simulink library "GFL_Lib"  (R2019b)
settings: Solver=VariableStepAuto  StartTime=0.0  StopTime=10.0  RelTol=1e-3
undefined symbols (not defined in the file or in its folder): Carm, Diff_CC_ki, Diff_CC_kp, fb, Ib2, Idcb, Ki_i, Ki_Wdiff_pu, Ki_Wtot_pu, Kp_i, Kp_Rvi_pu, Kp_Wdiff_pu, Kp_Wtot_pu, Lb, Lc_eq, Lc_pu, Lf_pu, Sb, Solver_Time_Step, Time_Step, Va0, Vb0, Vb1, Vb2, Vc0, Vdcb, Vm0, Vm0_d, Vm0_q, VSC01_id0, Vvsc0, wb, Zb
libraries: powerlib x90, Control_Lib x57, spsCurrentMeasurementLib x7, simulink x7, spsControlledCurrentSourceLib x6, $bdroot x5, Source_Lib x2, eeGeneralControl x2, powerlib_meascontrol x2, GFo_Lib x1
(part 2 of 5)

== system GFL_Lib/GFL IDEAL VSC ==
  note: do not modify this part if you use the update loaflow script
  note: Common Inputs
  note: Power part
  note: Measurements and normalization
  note: Control part
  dP_set (pu) : Inport
  dQ_set (pu) : Inport  Port=2
  1/Ib2 : Gain  Gain=1/Vb2
  1/Ib3 : Gain  Gain=1/Ib2
  Add : Sum
  Add1 : Sum
  Bridge_Model : Subsystem
  Bus01 : powerlib/Measurements/Three-Phase V-I Measurement  VoltageMeasurement=phase-to-ground  SetLabelV=off  LabelV=Vabc  Vpu=off  VpuLL=off  CurrentMeasurement=yes  SetLabelI=off  LabelI=Iabc  Ipu=off  Pbase=100e6  Vbase=500e3  OutputType=Complex  PhasorSimulation=off  PSBequivalent=0
  Control loops : Subsystem
  DC_Link : Source_Lib/DC_Link  Udc=Udcn  Pb=Pn  H_DC=H_DC
      settings: SourceProductName=VSC4SPS
  Output_Transformer : powerlib/Elements/Three-Phase Transformer (Two Windings)  Winding1Connection=Yg  Winding2Connection=Yg  CoreType=Three single-phase transformers  SetSaturation=off  Hysteresis=off  DataFile='hysteresis'  SetInitialFlux=off  Measurements=None  UNITS=pu  NominalPower=[Sn , fb]  Winding1=[Un1 , Rt_pu/2*(m^2), Lt_pu/2*(m^2)]  Winding2="[Un2*m ,  Rt_pu/2*(m^2), Lt_pu/2*(m^2)]"  Rm=Rm_pu  Lm=Lm_pu  L0=0.5  Saturation=[ 0,0 ; 0.0024,1.2 ; 1.0,1.52 ]  InitialFluxes=[ 0.8 , -0.8 , 0.7 ]  BreakLoop=off  DiscreteSolver=Trapezoidal iterative  DataType=off  TransfoNumber=1
  Pinit : Constant  Value=P0
  Source_For_LF : powerlib/Electrical Sources/Three-Phase Source  Commented=on  InternalConnection=Yg  VoltagePhases=off  Voltage=(690)*0.999921  PhaseAngle=3.7838  Voltage_phases=[25e3 25e3 25e3]/sqrt(3)  PhaseAngles_phases=[0 -120 +120]  Frequency=fb  NonIdealSource=off  SpecifyImpedance=off  Resistance=0  Inductance=0  ShortCircuitLevel=100e6  BaseVoltage=Un  XRratio=7  BusType=PQ  Pref=P0*Sb  Qref=Q0*Sb  Prefabc=[10e3, 10e3, 10e3]  Qrefabc=[0, 0, 0]  Qmin=-inf  Qmax=inf
  Transport Delay1 : TransportDelay  DelayTime=Output_Delay  InitialOutput=[Va0 Vb0 Vc0]
  Vvsc_init : Constant  Value=Q0
  mp3 : Gain  Gain=Vb1
  A : PMIOPort  Side=Right
  B : PMIOPort  Port=2  Side=Right
  C : PMIOPort  Port=3  Side=Right
  + : PMIOPort  Port=4  Side=Left
  - : PMIOPort  Port=5  Side=Left
  m : Outport  VectorParamsAs1DForOutWhenUnconnected=off
  wires:
  Bus01/2 -> [ig_meas]
  Transport Delay1/1 -> Bridge_Model/1(Uref)
  Bus01/1 -> [vg_meas]
  Add/1 -> Control loops/1(P_set)
  Control loops/2(m) -> m/1  "Control"
  mp3/1 -> Transport Delay1/1
  1/Ib3/1 -> Control loops/4(ig_abc_pu)  "ig_pu"
  1/Ib2/1 -> Control loops/3(vg_abc_pu)  "vg_pu"
  [vg_meas] -> 1/Ib2/1
  Control loops/1(vm_abc_ref_pu) -> mp3/1
  Add1/1 -> Control loops/2(Q_set)
  dP_set (pu)/1 -> Add/1
  Pinit/1 -> Add/2
  Vvsc_init/1 -> Add1/2
  dQ_set (pu)/1 -> Add1/1
  [ig_meas] -> 1/Ib3/1
  connections:
  Bridge_Model/LConn2 -- DC_Link/RConn3 -- -/RConn1
  Bridge_Model/LConn1 -- DC_Link/RConn1 -- +/RConn1
  Output_Transformer/RConn3 -- Bus01/LConn3
  Output_Transformer/LConn2 -- Bridge_Model/RConn2
  Output_Transformer/RConn1 -- Bus01/LConn1
  Output_Transformer/RConn2 -- Bus01/LConn2
  Output_Transformer/LConn1 -- Bridge_Model/RConn1
  Output_Transformer/LConn3 -- Bridge_Model/RConn3
  Bus01/RConn1 -- Source_For_LF/RConn1 -- A/RConn1
  Bus01/RConn3 -- Source_For_LF/RConn3 -- C/RConn1
  Bus01/RConn2 -- Source_For_LF/RConn2 -- B/RConn1

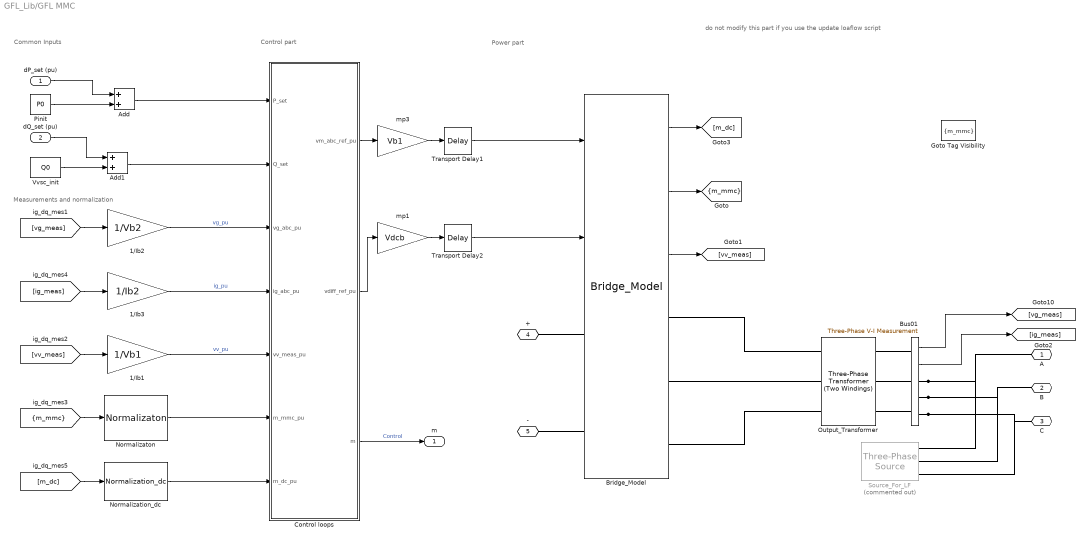
== system GFL_Lib/GFL MMC ==
  note: Common Inputs
  note: Control part
  note: Power part
  note: do not modify this part if you use the update loaflow script
  note: Measurements and normalization
  dP_set (pu) : Inport
  dQ_set (pu) : Inport  Port=2
  1/Ib1 : Gain  Gain=1/Vb1
  1/Ib2 : Gain  Gain=1/Vb2
  1/Ib3 : Gain  Gain=1/Ib2
  Add : Sum
  Add1 : Sum
  Bridge_Model : $bdroot/GFM_VC MMC/Bridge_Model  SystemSampleTime=-1  Latency=0  AutoFrameSizeCalculation=off
  Bus01 : powerlib/Measurements/Three-Phase V-I Measurement  VoltageMeasurement=phase-to-ground  SetLabelV=off  LabelV=Vabc  Vpu=off  VpuLL=off  CurrentMeasurement=yes  SetLabelI=off  LabelI=Iabc  Ipu=off  Pbase=100e6  Vbase=500e3  OutputType=Complex  PhasorSimulation=off  PSBequivalent=0
  Control loops : Subsystem
  Goto Tag Visibility : GotoTagVisibility  GotoTag=m_mmc
  Normalization_dc : $bdroot/GFM_VC MMC/Normalization_dc  SystemSampleTime=-1  Latency=0  AutoFrameSizeCalculation=off
  Normalizaton : $bdroot/GFM_VC MMC/Normalizaton  SystemSampleTime=-1  Latency=0  AutoFrameSizeCalculation=off
  Output_Transformer : powerlib/Elements/Three-Phase Transformer (Two Windings)  Winding1Connection=Yg  Winding2Connection=Yg  CoreType=Three single-phase transformers  SetSaturation=off  Hysteresis=off  DataFile='hysteresis'  SetInitialFlux=off  Measurements=None  UNITS=pu  NominalPower=[Sn , fb]  Winding1=[Un1 , Rt_pu/2 , Lt_pu/2]  Winding2=[Un2 , Rt_pu/2 , Lt_pu/2]  Rm=Rm_pu  Lm=Lm_pu  L0=0.5  Saturation=[ 0,0 ; 0.0024,1.2 ; 1.0,1.52 ]  InitialFluxes=[ 0.8 , -0.8 , 0.7 ]  BreakLoop=off  DiscreteSolver=Trapezoidal iterative  DataType=off  TransfoNumber=1
  Pinit : Constant  Value=P0
  Source_For_LF : powerlib/Electrical Sources/Three-Phase Source  Commented=on  InternalConnection=Yg  VoltagePhases=off  Voltage=(400000)*1  PhaseAngle=9.4519e-16  Voltage_phases=[25e3 25e3 25e3]/sqrt(3)  PhaseAngles_phases=[0 -120 +120]  Frequency=fb  NonIdealSource=off  SpecifyImpedance=off  Resistance=0  Inductance=0  ShortCircuitLevel=100e6  BaseVoltage=Un  XRratio=7  BusType=PQ  Pref=P0*Sb  Qref=Q0*Sb  Prefabc=[10e3, 10e3, 10e3]  Qrefabc=[0, 0, 0]  Qmin=-inf  Qmax=inf
  Transport Delay1 : TransportDelay  DelayTime=Output_Delay  InitialOutput=[Va0 Vb0 Vc0]
  Transport Delay2 : TransportDelay  DelayTime=Output_Delay  InitialOutput=[Udcn/2 Udcn/2 Udcn/2]
  Vvsc_init : Constant  Value=Q0
  mp1 : Gain  Gain=Vdcb
  mp3 : Gain  Gain=Vb1
  A : PMIOPort  Side=Right
  B : PMIOPort  Port=2  Side=Right
  C : PMIOPort  Port=3  Side=Right
  + : PMIOPort  Port=4  Side=Left
  - : PMIOPort  Port=5  Side=Left
  m : Outport  VectorParamsAs1DForOutWhenUnconnected=off
  tag scope: m_mmc=scoped
  wires:
  Add/1 -> Control loops/1(P_set)
  Control loops/3(m) -> m/1  "Control"
  mp3/1 -> Transport Delay1/1
  Control loops/1(vm_abc_ref_pu) -> mp3/1
  Add1/1 -> Control loops/2(Q_set)
  dP_set (pu)/1 -> Add/1
  Pinit/1 -> Add/2
  Vvsc_init/1 -> Add1/2
  dQ_set (pu)/1 -> Add1/1
  Bridge_Model/2 -> [m_mmc]
  Transport Delay2/1 -> Bridge_Model/2
  Bridge_Model/3 -> [vv_meas]
  Bus01/2 -> [ig_meas]
  Bridge_Model/1 -> [m_dc]
  Bus01/1 -> [vg_meas]
  Transport Delay1/1 -> Bridge_Model/1
  1/Ib1/1 -> Control loops/5(vv_meas_pu)  "vv_pu"
  Normalization_dc/1 -> Control loops/7(m_dc_pu)
  [vg_meas] -> 1/Ib2/1
  Normalizaton/1 -> Control loops/6(m_mmc_pu)
  [m_mmc] -> Normalizaton/1
  [vv_meas] -> 1/Ib1/1
  [ig_meas] -> 1/Ib3/1
  [m_dc] -> Normalization_dc/1
  1/Ib3/1 -> Control loops/4(ig_abc_pu)  "ig_pu"
  1/Ib2/1 -> Control loops/3(vg_abc_pu)  "vg_pu"
  mp1/1 -> Transport Delay2/1
  Control loops/2(vdiff_ref_pu) -> mp1/1
  connections:
  Bus01/RConn3 -- Source_For_LF/RConn3 -- C/RConn1
  Bus01/RConn1 -- Source_For_LF/RConn1 -- A/RConn1
  Bus01/RConn2 -- Source_For_LF/RConn2 -- B/RConn1
  Bridge_Model/RConn2 -- Output_Transformer/LConn2
  Output_Transformer/RConn1 -- Bus01/LConn1
  +/RConn1 -- Bridge_Model/LConn1
  -/RConn1 -- Bridge_Model/LConn2
  Output_Transformer/RConn2 -- Bus01/LConn2
  Bridge_Model/RConn1 -- Output_Transformer/LConn1
  Output_Transformer/RConn3 -- Bus01/LConn3
  Bridge_Model/RConn3 -- Output_Transformer/LConn3

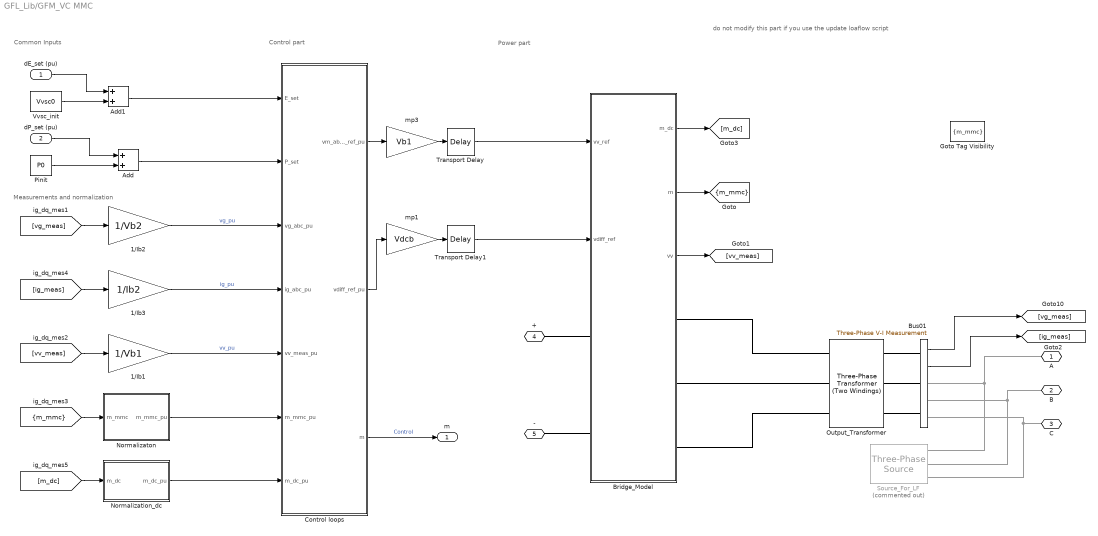
== system GFL_Lib/GFM_VC MMC ==
  note: do not modify this part if you use the update loaflow script
  note: Common Inputs
  note: Power part
  note: Measurements and normalization
  note: Control part
  dE_set (pu) : Inport
  dP_set (pu) : Inport  Port=2
  1/Ib1 : Gain  Gain=1/Vb1
  1/Ib2 : Gain  Gain=1/Vb2
  1/Ib3 : Gain  Gain=1/Ib2
  Add : Sum
  Add1 : Sum
  Bridge_Model : Subsystem
  Bus01 : powerlib/Measurements/Three-Phase V-I Measurement  VoltageMeasurement=phase-to-ground  SetLabelV=off  LabelV=Vabc  Vpu=off  VpuLL=off  CurrentMeasurement=yes  SetLabelI=off  LabelI=Iabc  Ipu=off  Pbase=100e6  Vbase=500e3  OutputType=Complex  PhasorSimulation=off  PSBequivalent=0
  Control loops : Subsystem
  Goto Tag Visibility : GotoTagVisibility  GotoTag=m_mmc
  Normalization_dc : Subsystem
  Normalizaton : Subsystem
  Output_Transformer : powerlib/Elements/Three-Phase Transformer (Two Windings)  Winding1Connection=Yg  Winding2Connection=Yg  CoreType=Three single-phase transformers  SetSaturation=off  Hysteresis=off  DataFile='hysteresis'  SetInitialFlux=off  Measurements=None  UNITS=pu  NominalPower=[Sn , fb]  Winding1=[Un1 , Rt_pu/2 , Lt_pu/2]  Winding2=[Un2 , Rt_pu/2 , Lt_pu/2]  Rm=Rm_pu  Lm=Lm_pu  L0=0.5  Saturation=[ 0,0 ; 0.0024,1.2 ; 1.0,1.52 ]  InitialFluxes=[ 0.8 , -0.8 , 0.7 ]  BreakLoop=off  DiscreteSolver=Trapezoidal iterative  DataType=off  TransfoNumber=1
  Pinit : Constant  Value=P0
  Source_For_LF : powerlib/Electrical Sources/Three-Phase Source  Commented=on  InternalConnection=Yg  VoltagePhases=off  Voltage=(400000)*1  PhaseAngle=9.4519e-16  Voltage_phases=[25e3 25e3 25e3]/sqrt(3)  PhaseAngles_phases=[0 -120 +120]  Frequency=fb  NonIdealSource=off  SpecifyImpedance=off  Resistance=0  Inductance=0  ShortCircuitLevel=100e6  BaseVoltage=Un  XRratio=7  BusType=PQ  Pref=P0*Sb  Qref=Q0*Sb  Prefabc=[10e3, 10e3, 10e3]  Qrefabc=[0, 0, 0]  Qmin=-inf  Qmax=inf
  Transport Delay : TransportDelay  DelayTime=Output_Delay  InitialOutput=[Va0 Vb0 Vc0]
  Transport Delay1 : TransportDelay  DelayTime=Output_Delay  InitialOutput=[Udcn/2 Udcn/2 Udcn/2]
  Vvsc_init : Constant  Value=Vvsc0
  mp1 : Gain  Gain=Vdcb
  mp3 : Gain  Gain=Vb1
  A : PMIOPort  Side=Right
  B : PMIOPort  Port=2  Side=Right
  C : PMIOPort  Port=3  Side=Right
  + : PMIOPort  Port=4  Side=Left
  - : PMIOPort  Port=5  Side=Left
  m : Outport  VectorParamsAs1DForOutWhenUnconnected=off
  tag scope: m_mmc=scoped
  wires:
  Add/1 -> Control loops/2(P_set)
  Control loops/3(m) -> m/1  "Control"
  mp3/1 -> Transport Delay/1
  1/Ib3/1 -> Control loops/4(ig_abc_pu)  "ig_pu"
  1/Ib2/1 -> Control loops/3(vg_abc_pu)  "vg_pu"
  [vg_meas] -> 1/Ib2/1
  Control loops/1(vm_abc_ref_pu) -> mp3/1
  Add1/1 -> Control loops/1(E_set)
  Transport Delay/1 -> Bridge_Model/1(vv_ref)
  dP_set (pu)/1 -> Add/1
  Pinit/1 -> Add/2
  Vvsc_init/1 -> Add1/2
  Bus01/1 -> [vg_meas]
  dE_set (pu)/1 -> Add1/1
  Bus01/2 -> [ig_meas]
  [ig_meas] -> 1/Ib3/1
  Control loops/2(vdiff_ref_pu) -> mp1/1
  mp1/1 -> Transport Delay1/1
  Transport Delay1/1 -> Bridge_Model/2(vdiff_ref)
  Bridge_Model/3(vv) -> [vv_meas]
  [vv_meas] -> 1/Ib1/1
  1/Ib1/1 -> Control loops/5(vv_meas_pu)  "vv_pu"
  [m_mmc] -> Normalizaton/1(m_mmc)
  Normalizaton/1(m_mmc_pu) -> Control loops/6(m_mmc_pu)
  Bridge_Model/1(m_dc) -> [m_dc]
  Normalization_dc/1(m_dc_pu) -> Control loops/7(m_dc_pu)
  [m_dc] -> Normalization_dc/1(m_dc)
  Bridge_Model/2(m) -> [m_mmc]
  connections:
  Output_Transformer/RConn1 -- Bus01/LConn1
  Output_Transformer/RConn2 -- Bus01/LConn2
  Output_Transformer/RConn3 -- Bus01/LConn3
  Source_For_LF/RConn2 -- B/RConn1 -- Bus01/RConn2
  Source_For_LF/RConn1 -- A/RConn1 -- Bus01/RConn1
  Source_For_LF/RConn3 -- C/RConn1 -- Bus01/RConn3
  Bridge_Model/RConn1 -- Output_Transformer/LConn1
  Bridge_Model/RConn2 -- Output_Transformer/LConn2
  Bridge_Model/RConn3 -- Output_Transformer/LConn3
  +/RConn1 -- Bridge_Model/LConn1
  -/RConn1 -- Bridge_Model/LConn2

== system GFL_Lib/Mean Model 2-Level L-filter with DC Link ==
  note: Control part
  note: Measurements and normalization
  note: Power part
  note: Common Inputs
  note: do not modify this part if you use the update loaflow script
  dP_set (pu) : Inport
  dQ_set (pu) : Inport  Port=2
  1/Ib2 : Gain  Gain=1/Vb2
  1/Ib3 : Gain  Gain=1/Ib2
  Add : Sum
  Add1 : Sum
  Bridge_Model : Subsystem
  Bus01 : powerlib/Measurements/Three-Phase V-I Measurement  VoltageMeasurement=phase-to-ground  SetLabelV=off  LabelV=Vabc  Vpu=off  VpuLL=off  CurrentMeasurement=yes  SetLabelI=off  LabelI=Iabc  Ipu=off  Pbase=100e6  Vbase=500e3  OutputType=Complex  PhasorSimulation=off  PSBequivalent=0
  Control loops : Subsystem
  DC_Link_1 : powerlib/Elements/Series RLC Branch  LConnTagsString=__new0  RConnTagsString=__new0  BranchType=C  Resistance=1  Inductance=1e-3  SetiL0=off  InitialCurrent=0  Capacitance=0.00039063  Setx0=on  InitialVoltage=Udcn/2  Measurements=None
  DC_Link_2 : powerlib/Elements/Series RLC Branch  LConnTagsString=__new0  RConnTagsString=__new0  BranchType=C  Resistance=1  Inductance=1e-3  SetiL0=off  InitialCurrent=0  Capacitance=0.00039063  Setx0=on  InitialVoltage=Udcn/2  Measurements=None
  Delay : Delay  DelayLength=1  InitialCondition=[Va0 Vb0 Vc0]  SampleTime=Solver_Time_Step
  Ground : powerlib/Elements/Ground  LConnTagsString=a
  Output_Transformer : powerlib/Elements/Three-Phase Transformer (Two Windings)  Winding1Connection=Yg  Winding2Connection=Yg  CoreType=Three single-phase transformers  SetSaturation=off  Hysteresis=off  DataFile='hysteresis'  SetInitialFlux=off  Measurements=None  UNITS=pu  NominalPower=[Sn , fb]  Winding1=[Un1 , Rt_pu/2*(m^2), Lt_pu/2*(m^2)]  Winding2="[Un2*m ,  Rt_pu/2*(m^2), Lt_pu/2*(m^2)]"  Rm=Rm_pu  Lm=Lm_pu  L0=0.5  Saturation=[ 0,0 ; 0.0024,1.2 ; 1.0,1.52 ]  InitialFluxes=[ 0.8 , -0.8 , 0.7 ]  BreakLoop=off  DiscreteSolver=Trapezoidal iterative  DataType=off  TransfoNumber=1
  Pinit : Constant  Value=P0
  Source_For_LF : powerlib/Electrical Sources/Three-Phase Source  Commented=on  InternalConnection=Yg  VoltagePhases=off  Voltage=(400000)*1.01081  PhaseAngle=0.4912  Voltage_phases=[25e3 25e3 25e3]/sqrt(3)  PhaseAngles_phases=[0 -120 +120]  Frequency=fb  NonIdealSource=off  SpecifyImpedance=off  Resistance=0  Inductance=0  ShortCircuitLevel=100e6  BaseVoltage=Un  XRratio=7  BusType=PQ  Pref=P0*Sb  Qref=Q0*Sb  Prefabc=[10e3, 10e3, 10e3]  Qrefabc=[0, 0, 0]  Qmin=-inf  Qmax=inf
  Vvsc_init : Constant  Value=Q0
  mp3 : Gain  Gain=Vb1
  A : PMIOPort  Side=Right
  B : PMIOPort  Port=2  Side=Right
  C : PMIOPort  Port=3  Side=Right
  A1 : PMIOPort  Port=4  Side=Left
  A2 : PMIOPort  Port=5  Side=Left
  m : Outport  VectorParamsAs1DForOutWhenUnconnected=off
  wires:
  [ig_meas] -> 1/Ib3/1
  dQ_set (pu)/1 -> Add1/1
  Vvsc_init/1 -> Add1/2
  Pinit/1 -> Add/2
  dP_set (pu)/1 -> Add/1
  Add1/1 -> Control loops/2(Q_set)
  Control loops/1(vm_abc_ref_pu) -> mp3/1
  [vg_meas] -> 1/Ib2/1
  1/Ib2/1 -> Control loops/3(vg_abc_pu)  "vg_pu"
  1/Ib3/1 -> Control loops/4(ig_abc_pu)  "ig_pu"
  mp3/1 -> Delay/1
  Control loops/2(m) -> m/1  "Control"
  Add/1 -> Control loops/1(P_set)
  Bus01/1 -> [vg_meas]
  Delay/1 -> Bridge_Model/1(Uref)
  Bus01/2 -> [ig_meas]
  connections:
  B/RConn1 -- Source_For_LF/RConn2 -- Bus01/RConn2
  C/RConn1 -- Source_For_LF/RConn3 -- Bus01/RConn3
  A/RConn1 -- Source_For_LF/RConn1 -- Bus01/RConn1
  Output_Transformer/LConn3 -- Bridge_Model/RConn3
  Output_Transformer/LConn1 -- Bridge_Model/RConn1
  Output_Transformer/RConn2 -- Bus01/LConn2
  Output_Transformer/RConn1 -- Bus01/LConn1
  Output_Transformer/LConn2 -- Bridge_Model/RConn2
  Output_Transformer/RConn3 -- Bus01/LConn3
  DC_Link_1/LConn1 -- A1/RConn1 -- Bridge_Model/LConn1
  DC_Link_2/RConn1 -- Bridge_Model/LConn2 -- A2/RConn1
  DC_Link_1/RConn1 -- DC_Link_2/LConn1 -- Ground/LConn1

== system GFL_Lib/Mean Model 2-Level L-filter_old ==
  note: Control part
  note: Measurements and normalization
  note: Power part
  note: Common Inputs
  note: do not modify this part if you use the update loaflow script
  dP_set (pu) : Inport
  dQ_set (pu) : Inport  Port=2
  1/Ib2 : Gain  Gain=1/Vb2
  1/Ib3 : Gain  Gain=1/Ib2
  Add : Sum
  Add1 : Sum
  Bridge_Model : Subsystem
  Bus01 : powerlib/Measurements/Three-Phase V-I Measurement  VoltageMeasurement=phase-to-ground  SetLabelV=off  LabelV=Vabc  Vpu=off  VpuLL=off  CurrentMeasurement=yes  SetLabelI=off  LabelI=Iabc  Ipu=off  Pbase=100e6  Vbase=500e3  OutputType=Complex  PhasorSimulation=off  PSBequivalent=0
  Control loops : Subsystem
  DC_Link : Source_Lib/DC_Link  Udc=Udcn  Pb=Pn  H_DC=H_DC
      settings: SourceProductName=VSC4SPS
  Delay : Delay  DelayLength=1  InitialCondition=[Va0 Vb0 Vc0]  SampleTime=Output_Delay/1.5
  Output_Transformer : powerlib/Elements/Three-Phase Transformer (Two Windings)  Winding1Connection=Yg  Winding2Connection=Yg  CoreType=Three single-phase transformers  SetSaturation=off  Hysteresis=off  DataFile='hysteresis'  SetInitialFlux=off  Measurements=None  UNITS=pu  NominalPower=[Sn , fb]  Winding1=[Un1 , Rt_pu/2*(m^2), Lt_pu/2*(m^2)]  Winding2="[Un2*m ,  Rt_pu/2*(m^2), Lt_pu/2*(m^2)]"  Rm=Rm_pu  Lm=Lm_pu  L0=0.5  Saturation=[ 0,0 ; 0.0024,1.2 ; 1.0,1.52 ]  InitialFluxes=[ 0.8 , -0.8 , 0.7 ]  BreakLoop=off  DiscreteSolver=Trapezoidal iterative  DataType=off  TransfoNumber=1
  Pinit : Constant  Value=P0
  Source_For_LF : powerlib/Electrical Sources/Three-Phase Source  Commented=on  InternalConnection=Yg  VoltagePhases=off  Voltage=(400000)*1.01081  PhaseAngle=0.4912  Voltage_phases=[25e3 25e3 25e3]/sqrt(3)  PhaseAngles_phases=[0 -120 +120]  Frequency=fb  NonIdealSource=off  SpecifyImpedance=off  Resistance=0  Inductance=0  ShortCircuitLevel=100e6  BaseVoltage=Un  XRratio=7  BusType=PQ  Pref=P0*Sb  Qref=Q0*Sb  Prefabc=[10e3, 10e3, 10e3]  Qrefabc=[0, 0, 0]  Qmin=-inf  Qmax=inf
  Vvsc_init : Constant  Value=Q0
  mp3 : Gain  Gain=Vb1
  A : PMIOPort  Side=Right
  B : PMIOPort  Port=2  Side=Right
  C : PMIOPort  Port=3  Side=Right
  + : PMIOPort  Port=4  Side=Left
  0 : PMIOPort  Port=5  Side=Left
  - : PMIOPort  Port=6  Side=Left
  m : Outport  VectorParamsAs1DForOutWhenUnconnected=off
  wires:
  [ig_meas] -> 1/Ib3/1
  dQ_set (pu)/1 -> Add1/1
  Vvsc_init/1 -> Add1/2
  Pinit/1 -> Add/2
  dP_set (pu)/1 -> Add/1
  Add1/1 -> Control loops/2(Q_set)
  Control loops/1(vm_abc_ref_pu) -> mp3/1
  [vg_meas] -> 1/Ib2/1
  1/Ib2/1 -> Control loops/3(vg_abc_pu)  "vg_pu"
  1/Ib3/1 -> Control loops/4(ig_abc_pu)  "ig_pu"
  mp3/1 -> Delay/1
  Control loops/2(m) -> m/1  "Control"
  Add/1 -> Control loops/1(P_set)
  Bus01/1 -> [vg_meas]
  Delay/1 -> Bridge_Model/1(Uref)
  Bus01/2 -> [ig_meas]
  connections:
  B/RConn1 -- Source_For_LF/RConn2 -- Bus01/RConn2
  C/RConn1 -- Source_For_LF/RConn3 -- Bus01/RConn3
  A/RConn1 -- Source_For_LF/RConn1 -- Bus01/RConn1
  Output_Transformer/LConn3 -- Bridge_Model/RConn3
  Output_Transformer/LConn1 -- Bridge_Model/RConn1
  Output_Transformer/RConn2 -- Bus01/LConn2
  Output_Transformer/RConn1 -- Bus01/LConn1
  Output_Transformer/LConn2 -- Bridge_Model/RConn2
  Output_Transformer/RConn3 -- Bus01/LConn3
  DC_Link/RConn1 -- +/RConn1 -- Bridge_Model/LConn1
  DC_Link/RConn3 -- Bridge_Model/LConn2 -- -/RConn1
  0/RConn1 -- DC_Link/RConn2

== system GFL_Lib/Mean Model 2-Level L-filter_sav ==
  note: do not modify this part if you use the update loaflow script
  note: Transformer
  note: Common Inputs
  note: Power part
  note: Measurements and normalization
  note: Control part
  dQ_set (pu) : Inport
  dP_set (pu) : Inport  Port=2
  1/Ib2 : Gain  Gain=1/Vb2
  1/Ib3 : Gain  Gain=1/Ib2
  Add : Sum
  Add1 : Sum
  Bus Creator : BusCreator  Inputs=3
  Bus01 : powerlib/Measurements/Three-Phase V-I Measurement  VoltageMeasurement=phase-to-ground  SetLabelV=off  LabelV=Vabc  Vpu=off  VpuLL=off  CurrentMeasurement=yes  SetLabelI=off  LabelI=Iabc  Ipu=off  Pbase=100e6  Vbase=500e3  OutputType=Complex  PhasorSimulation=off  PSBequivalent=0
  Control loops : Subsystem
  DC Voltage Source : powerlib/Electrical Sources/DC Voltage Source  Amplitude=Udcn  Measurements=Voltage
  Load Flow Bus : powerlib/Measurements/Load Flow Bus  LConnTagsString=a  Phases=single  Connectors=on one side  ID=Mean Model 2-Level L-filter_sav  Vbase=Un2  Vref=1.0015  Vangle=0.56166  VLF=1.002  VLFb=1  VLFc=1  angleLF=0.5617  angleLFb=0  angleLFc=0
  Mean_Model : Subsystem
  Memory1 : Memory  InitialCondition=[Va0 Vb0 Vc0]
  Output_Transformer : powerlib/Elements/Three-Phase Transformer (Two Windings)  Winding1Connection=Yg  Winding2Connection=Yg  CoreType=Three single-phase transformers  SetSaturation=off  Hysteresis=off  DataFile='hysteresis'  SetInitialFlux=off  Measurements=None  UNITS=pu  NominalPower=[Sn , fb]  Winding1=[Un1 , Rt_pu/2 , Lt_pu/2]  Winding2=[Un2 , Rt_pu/2 , Lt_pu/2]  Rm=Rm_pu  Lm=Lm_pu  L0=0.5  Saturation=[ 0,0 ; 0.0024,1.2 ; 1.0,1.52 ]  InitialFluxes=[ 0.8 , -0.8 , 0.7 ]  BreakLoop=off  DiscreteSolver=Trapezoidal iterative  DataType=off  TransfoNumber=1
  Pinit : Constant  Value=P0
  Source_For_LF : powerlib/Electrical Sources/Three-Phase Source  Commented=on  InternalConnection=Yg  VoltagePhases=off  Voltage=(400)*1.00151  PhaseAngle=0.56166  Voltage_phases=[25e3 25e3 25e3]/sqrt(3)  PhaseAngles_phases=[0 -120 +120]  Frequency=fb  NonIdealSource=off  SpecifyImpedance=off  Resistance=0  Inductance=0  ShortCircuitLevel=100e6  BaseVoltage=Un  XRratio=7  BusType=PQ  Pref=P0*Sb  Qref=Q0*Sb  Prefabc=[10e3, 10e3, 10e3]  Qrefabc=[0, 0, 0]  Qmin=-inf  Qmax=inf
  Vvsc_init : Constant  Value=Q0
  mp3 : Gain  Gain=Vb1
  A : PMIOPort  Side=Right
  B : PMIOPort  Port=2  Side=Right
  C : PMIOPort  Port=3  Side=Right
  m : Outport  VectorParamsAs1DForOutWhenUnconnected=off
  wires:
  Add/1 -> Control loops/1(P_set)
  Control loops/2(m) -> Bus Creator/1  "Control"
  mp3/1 -> Memory1/1
  1/Ib3/1 -> Bus Creator/3, Control loops/4(ig_abc_pu)  "ig_pu"
  1/Ib2/1 -> Bus Creator/2, Control loops/3(vg_abc_pu)  "vg_pu"
  Bus Creator/1 -> m/1
  [vg_meas] -> 1/Ib2/1
  Control loops/1(vm_abc_ref_pu) -> mp3/1
  Add1/1 -> Control loops/2(Q_set)
  Memory1/1 -> Mean_Model/1(Uref)
  dP_set (pu)/1 -> Add/1
  Pinit/1 -> Add/2
  Vvsc_init/1 -> Add1/2
  Bus01/1 -> [vg_meas]
  dQ_set (pu)/1 -> Add1/1
  Bus01/2 -> [ig_meas]
  [ig_meas] -> 1/Ib3/1
  connections:
  DC Voltage Source/LConn1 -- Mean_Model/LConn2
  Output_Transformer/RConn1 -- Bus01/LConn1
  Output_Transformer/RConn2 -- Bus01/LConn2
  DC Voltage Source/RConn1 -- Mean_Model/LConn1
  Output_Transformer/RConn3 -- Bus01/LConn3
  Source_For_LF/RConn2 -- B/RConn1 -- Bus01/RConn2
  Mean_Model/RConn1 -- Output_Transformer/LConn1
  Mean_Model/RConn2 -- Output_Transformer/LConn2
  Mean_Model/RConn3 -- Output_Transformer/LConn3
  Source_For_LF/RConn1 -- Load Flow Bus/LConn1 -- A/RConn1 -- Bus01/RConn1
  Source_For_LF/RConn3 -- C/RConn1 -- Bus01/RConn3

== system GFL_Lib/Mean Model 2-Level LCL-filter [under construction] ==
  note: Common Inputs
  note: Power part
  note: Measurements and normalization
  note: Control part
  dQ_set (pu) : Inport
  dP_set (pu) : Inport  Port=2
  1/Ib2 : Gain  Gain=1/Vb2
  1/Ib3 : Gain  Gain=1/Ib2
  Add : Sum
  Add1 : Sum
  Bus Creator : BusCreator  Inputs=3
  Bus01 : powerlib/Measurements/Three-Phase V-I Measurement  VoltageMeasurement=phase-to-ground  SetLabelV=off  LabelV=Vabc  Vpu=off  VpuLL=off  CurrentMeasurement=yes  SetLabelI=off  LabelI=Iabc  Ipu=off  Pbase=100e6  Vbase=500e3  OutputType=Complex  PhasorSimulation=off  PSBequivalent=0
  Bus1 : powerlib/Measurements/Three-Phase V-I Measurement  VoltageMeasurement=phase-to-ground  SetLabelV=off  LabelV=Vabc  Vpu=off  VpuLL=off  CurrentMeasurement=no  SetLabelI=off  LabelI=Iabc  Ipu=off  Pbase=100e6  Vbase=500e3  OutputType=Complex  PhasorSimulation=off  PSBequivalent=0
  Bus2 : powerlib/Measurements/Three-Phase V-I Measurement  VoltageMeasurement=no  SetLabelV=off  LabelV=Vabc  Vpu=off  VpuLL=off  CurrentMeasurement=yes  SetLabelI=off  LabelI=Iabc  Ipu=off  Pbase=100e6  Vbase=500e3  OutputType=Complex  PhasorSimulation=off  PSBequivalent=0
  Control loops : Subsystem
  DC Voltage Source : powerlib/Electrical Sources/DC Voltage Source  Amplitude=Udcn  Measurements=Voltage
  Load Flow Bus : powerlib/Measurements/Load Flow Bus  LConnTagsString=a  Phases=single  Connectors=on one side  ID=|  Vbase=Un2  Vref=1.0015  Vangle=0.56166  VLF=1.002  VLFb=1  VLFc=1  angleLF=0.5617  angleLFb=0  angleLFc=0
      | Mean Model
      | 2-Level LCL-filter [under construction]
  Mean_model : Subsystem
  Memory1 : Memory  InitialCondition=[Va0 Vb0 Vc0]
  Output_Filter : GFo_Lib/Mean Model 2-Level LCL-filter/Output_Filter
      settings: SourceProductName=VSC4SPS
  Output_Transformer : powerlib/Elements/Three-Phase Transformer (Two Windings)  Winding1Connection=Yg  Winding2Connection=Yg  CoreType=Three single-phase transformers  SetSaturation=off  Hysteresis=off  DataFile='hysteresis'  SetInitialFlux=off  Measurements=None  UNITS=pu  NominalPower=[Sn , fb]  Winding1=[Un1 , Rt_pu/2 , Lt_pu/2]  Winding2=[Un2 , Rt_pu/2 , Lt_pu/2]  Rm=Rm_pu  Lm=Lm_pu  L0=0.5  Saturation=[ 0,0 ; 0.0024,1.2 ; 1.0,1.52 ]  InitialFluxes=[-1.0109960716468 0.506091473811006 0.504904597835851]  BreakLoop=off  DiscreteSolver=Trapezoidal iterative  DataType=off  TransfoNumber=1
  Pinit : Constant  Value=P0
  Source_For_LF : powerlib/Electrical Sources/Three-Phase Source  Commented=on  InternalConnection=Yg  VoltagePhases=off  Voltage=(400)*1.00151  PhaseAngle=0.56166  Voltage_phases=[25e3 25e3 25e3]/sqrt(3)  PhaseAngles_phases=[0 -120 +120]  Frequency=fb  NonIdealSource=off  SpecifyImpedance=off  Resistance=0  Inductance=0  ShortCircuitLevel=100e6  BaseVoltage=Un  XRratio=7  BusType=PQ  Pref=P0*Sb  Qref=Q0*Sb  Prefabc=[10e3, 10e3, 10e3]  Qrefabc=[0, 0, 0]  Qmin=-inf  Qmax=inf
  Vvsc_init : Constant  Value=Q0
  mp3 : Gain  Gain=Vb1
  A : PMIOPort  Side=Right
  B : PMIOPort  Port=2  Side=Right
  C : PMIOPort  Port=3  Side=Right
  m : Outport  VectorParamsAs1DForOutWhenUnconnected=off
  wires:
  Add/1 -> Control loops/1(P_set)
  Control loops/2(m) -> Bus Creator/1  "Control"
  mp3/1 -> Memory1/1
  1/Ib3/1 -> Bus Creator/3, Control loops/4(ig_abc_pu)  "ig_pu"
  1/Ib2/1 -> Bus Creator/2, Control loops/3(vg_abc_pu)  "vg_pu"
  Bus Creator/1 -> m/1
  [vg_meas] -> 1/Ib2/1
  Control loops/1(vm_abc_ref_pu) -> mp3/1
  Add1/1 -> Control loops/2(Q_set)
  Memory1/1 -> Mean_model/1(Uref)
  dP_set (pu)/1 -> Add/1
  Pinit/1 -> Add/2
  Vvsc_init/1 -> Add1/2
  Bus01/1 -> [vg_meas]
  dQ_set (pu)/1 -> Add1/1
  Bus01/2 -> [ig_meas]
  [ig_meas] -> 1/Ib3/1
  Bus1/1 -> [eg_meas]
  Bus2/1 -> [is_meas]
  connections:
  DC Voltage Source/LConn1 -- Mean_model/LConn2
  Bus01/LConn1 -- Output_Transformer/RConn1
  Bus01/LConn2 -- Output_Transformer/RConn2
  DC Voltage Source/RConn1 -- Mean_model/LConn1
  Bus01/LConn3 -- Output_Transformer/RConn3
  Source_For_LF/RConn2 -- B/RConn1 -- Bus01/RConn2
  Source_For_LF/RConn1 -- Load Flow Bus/LConn1 -- A/RConn1 -- Bus01/RConn1
  Source_For_LF/RConn3 -- C/RConn1 -- Bus01/RConn3
  Bus1/LConn1 -- Output_Filter/RConn1
  Bus1/LConn2 -- Output_Filter/RConn2
  Bus1/LConn3 -- Output_Filter/RConn3
  Output_Transformer/LConn1 -- Bus1/RConn1
  Output_Transformer/LConn2 -- Bus1/RConn2
  Output_Transformer/LConn3 -- Bus1/RConn3
  Mean_model/RConn2 -- Bus2/LConn2
  Mean_model/RConn3 -- Bus2/LConn3
  Mean_model/RConn1 -- Bus2/LConn1
  Bus2/RConn1 -- Output_Filter/LConn1
  Bus2/RConn2 -- Output_Filter/LConn2
  Bus2/RConn3 -- Output_Filter/LConn3

== system GFL_Lib/GFL IDEAL VSC/Bridge_Model ==
  Uref : Inport
  NOT1 : Logic  Operator=NOT  IconShape=distinctive  AllPortsSameDT=off  OutDataTypeStr=boolean
  Saturation : Saturate  UpperLimit=1  LowerLimit=-1
  Step : Step  Time=Output_Delay  SampleTime=0
  Terminator : Terminator
  Three-Phase Breaker2 : powerlib/Elements/Three-Phase Breaker  InitialState=open  SwitchA=on  SwitchB=on  SwitchC=on  SwitchTimes="[4/60  10/60]"  External=on  BreakerResistance=1e-5*Zb  SnubberResistance=1e6  SnubberCapacitance=inf  Measurements=None
  Three-Phase Breaker3 : powerlib/Elements/Three-Phase Breaker  InitialState=closed  SwitchA=on  SwitchB=on  SwitchC=on  SwitchTimes="[4/60  10/60]"  External=on  BreakerResistance=1e-6*Zb  SnubberResistance=1e6  SnubberCapacitance=inf  Measurements=None
  Three-Phase Source : powerlib/Electrical Sources/Three-Phase Source  InternalConnection=Yg  VoltagePhases=off  Voltage=Vm0*Un1  PhaseAngle=Theta_Vm0  Voltage_phases=[25e3 25e3 25e3]/sqrt(3)  PhaseAngles_phases=[0 -120 +120]  Frequency=fb  NonIdealSource=off  SpecifyImpedance=off  Resistance=0  Inductance=0  ShortCircuitLevel=100e6  BaseVoltage=VSC01_Un1  XRratio=7  BusType=swing  Pref=0.3  Qref=0  Prefabc=[10e3, 10e3, 10e3]  Qrefabc=[0, 0, 0]  Qmin=-Inf  Qmax=Inf
  Universal Bridge : powerlib/Power Electronics/Universal Bridge  Arms=3  SnubberResistance=1e5  SnubberCapacitance=inf  Device=Average-model based VSC  Ron=1e-3  Lon=0  ForwardVoltages="[  0  0  ]"  ForwardVoltage=0  GTOparameters=[ 10e-6 , 20e-6 ]  IGBTparameters=[ 1e-6 , 2e-6 ]  Measurements=None  Measurements_2=None  converterType=Rectifier
  Vdc : powerlib/Measurements/Voltage Measurement  PhasorSimulation=off  OutputType=Complex  PSBequivalent=0
  mp3 : Gain  Gain=2/Udcn
  PhA : PMIOPort  Side=Right
  PhB : PMIOPort  Port=2  Side=Right
  PhC : PMIOPort  Port=3  Side=Right
  Vdc+ : PMIOPort  Port=4  Side=Left
  Vdc- : PMIOPort  Port=5  Side=Left
  wires:
  Step/1 -> Three-Phase Breaker2/1, NOT1/1
  Saturation/1 -> Universal Bridge/1
  NOT1/1 -> Three-Phase Breaker3/1
  mp3/1 -> Saturation/1
  Uref/1 -> mp3/1
  Vdc/1 -> Terminator/1
  connections:
  Three-Phase Breaker3/RConn3 -- Three-Phase Source/RConn3
  Three-Phase Breaker3/RConn2 -- Three-Phase Source/RConn2
  Three-Phase Breaker3/RConn1 -- Three-Phase Source/RConn1
  Three-Phase Breaker2/RConn1 -- Universal Bridge/LConn1
  Three-Phase Breaker2/RConn2 -- Universal Bridge/LConn2
  Three-Phase Breaker2/RConn3 -- Universal Bridge/LConn3
  Three-Phase Breaker2/LConn1 -- Three-Phase Breaker3/LConn1 -- PhA/RConn1
  Three-Phase Breaker2/LConn2 -- Three-Phase Breaker3/LConn2 -- PhB/RConn1
  Three-Phase Breaker2/LConn3 -- Three-Phase Breaker3/LConn3 -- PhC/RConn1
  Vdc/LConn1 -- Universal Bridge/RConn1 -- Vdc+/RConn1
  Vdc/LConn2 -- Universal Bridge/RConn2 -- Vdc-/RConn1

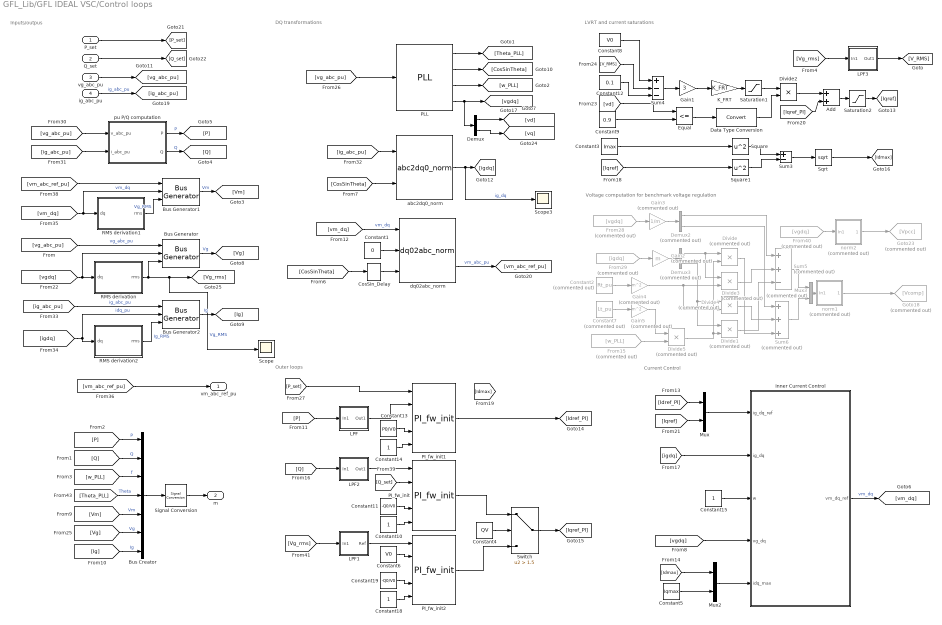
== system GFL_Lib/GFL IDEAL VSC/Control loops ==
  note: Inputs/outpus
  note: DQ transformations
  note: Current Control
  note: Outer loops
  note: LVRT and current saturations
  note: Voltage computation for benchmark voltage regulation
  P_set : Inport
  Q_set : Inport  Port=2
  vg_abc_pu : Inport  Port=3
  ig_abc_pu : Inport  Port=4
  " pu P/Q computation" : Subsystem  DialogController=POWERSYS.PowerSysDialog
  Add : Sum
  Bus Creator : BusCreator  Inputs=7
  Bus Generator : Control_Lib/Bus Generator  Gpu=0
      settings: SourceProductName=VSC4SPS
  Bus Generator1 : Control_Lib/Bus Generator  Gpu=0
      settings: SourceProductName=VSC4SPS
  Bus Generator2 : Control_Lib/Bus Generator  Gpu=0
      settings: SourceProductName=VSC4SPS
  Constant1 : Constant  Value=0
  Constant{10,14..15,18} (4 alike) : Constant
  Constant11 : Constant  Value=-Q0/V0
  Constant12 : Constant  Value=0.1
  Constant13 : Constant  Value=P0/V0
  Constant19 : Constant  Value=-Q0/V0
  Constant2 : Constant  Commented=on  Value=Rt_pu
  Constant3 : Constant  Value=Imax
  Constant4 : Constant  Value=QV
  Constant5 : Constant  Value=Iqmax
  Constant6 : Constant  Value=V0
  Constant7 : Constant  Commented=on  Value=Lt_pu
  Constant8 : Constant  Value=V0
  Constant9 : Constant  Value=0.9
  CosSin_Delay : Control_Lib/CosSin_Delay  dTheta=wb*Output_Delay
      settings: SourceProductName=VSC4SPS
  Data Type Conversion : DataTypeConversion
  Demux : Demux  Outputs=[1 1]
  Demux2 : Demux  Commented=on  Outputs=2
  Demux3 : Demux  Commented=on  Outputs=2
  Divide{,1,3..5} (5 alike) : Product  Commented=on  Inputs=**
  Divide2 : Product  Inputs=**
  Equal : RelationalOperator  Operator=<=  OutDataTypeStr=boolean  RndMeth=Simplest
  From15 : From  Commented=on  GotoTag=w_PLL
  From28 : From  Commented=on  GotoTag=vgdq
  From29 : From  Commented=on  GotoTag=igdq
  From40 : From  Commented=on  GotoTag=vgdq
  Gain1 : Gain  Gain=3
  Gain2 : Gain  Commented=on  Gain=m
  Gain3 : Gain  Commented=on  Gain=1/m
  Gain4 : Gain  Commented=on  Gain=m^2
  Gain5 : Gain  Commented=on  Gain=m^2
  Goto18 : Goto  Commented=on  GotoTag=Vcomp
  Goto23 : Goto  Commented=on  GotoTag=Vpcc
  Inner Current Control : Subsystem
  K_FRT : Gain  Gain=K_FRT
  LPF : Subsystem
  LPF1 : Subsystem
  LPF2 : Subsystem
  LPF3 : Subsystem
  Mux : Mux  Inputs=2
  Mux2 : Mux  Inputs=2
  Mux3 : Mux  Commented=on  Inputs=2
  PI_fw_init : Control_Lib/PI_fw_init  Kp=w_P/w_LPF  Ki=w_P
      settings: SourceProductName=VSC4SPS
  PI_fw_init1 : Control_Lib/PI_fw_init  Kp=w_P/w_LPF  Ki=w_P
      settings: SourceProductName=VSC4SPS
  PI_fw_init2 : Control_Lib/PI_fw_init  Kp=w_V/w_LPF  Ki=w_V
      settings: SourceProductName=VSC4SPS
  PLL : Control_Lib/PLL  fb=fb  wn_PLL=wn_PLL  zeta_PLL=zeta_PLL  Theta0=Theta0
      settings: SourceProductName=VSC4SPS
  RMS derivation : Subsystem
  RMS derivation1 : Subsystem
  RMS derivation2 : Subsystem
  Saturation1 : Saturate  UpperLimit=Imax  LowerLimit=-Imax
  Saturation2 : Saturate  UpperLimit=Imax  LowerLimit=-Imax
  Scope : Scope
  Scope3 : Scope
  Signal Conversion : SignalConversion  OverrideOpt=off
  Sqrt : Sqrt  SaturateOnIntegerOverflow=on
  Square : Math  Operator=square  SaturateOnIntegerOverflow=on
  Square1 : Math  Operator=square  SaturateOnIntegerOverflow=on
  Sum3 : Sum  Inputs=+-
  Sum4 : Sum  Inputs=+--
  Sum5 : Sum  Commented=on  Inputs=++-
  Sum6 : Sum  Commented=on  Inputs=+++
  Switch : Switch  Criteria=u2 > Threshold  Threshold=1.5
  abc2dq0_norm : Control_Lib/abc2dq0_norm  referenceAxisMode=Reference axis at 90 degrees behind phase_a  baseUpdateGain=1/sqrt(3)
      settings: SourceProductName=VSC4SPS
  dq02abc_norm : Control_Lib/dq02abc_norm  referenceAxisMode=Reference axis at 90 degrees behind phase_a  baseUpdateGain=sqrt(3)
      settings: SourceProductName=VSC4SPS
  norm1 : Subsystem  Commented=on
  norm2 : Subsystem  Commented=on
  vm_abc_ref_pu : Outport  VectorParamsAs1DForOutWhenUnconnected=off
  m : Outport  Port=2  VectorParamsAs1DForOutWhenUnconnected=off
  wires:
  Constant6/1 -> PI_fw_init2/2
  PI_fw_init2/1 -> Switch/3
  Constant14/1 -> PI_fw_init1/5
  Constant13/1 -> PI_fw_init1/4
  [Vg_rms] -> LPF3/1(In1)
  LPF3/1(Out1) -> [V_RMS]
  CosSin_Delay/1 -> dq02abc_norm/3
  [Theta_PLL] -> Bus Creator/4  "Theta"
  RMS derivation/1(rms) -> Bus Generator/3, [Vg_rms], Scope/1  "Vg_RMS"
  [vgdq] -> Bus Generator/2, RMS derivation/1(dq)
  Demux/2 -> [vq]
  Demux/1 -> [vd]
  PLL/4 -> [vgdq], Demux/1
  norm2/1(Out1) -> Goto23/1
  From40/1 -> norm2/1(In1)
  Gain4/1 -> Divide3/2, Divide4/2
  Gain5/1 -> Divide5/1
  Gain2/1 -> Demux3/1
  From29/1 -> Gain2/1
  [Q_set] -> PI_fw_init/2
  [vgdq] -> Inner Current Control/4(vg_dq)
  [vm_abc_ref_pu] -> Bus Generator1/1
  [vm_abc_ref_pu] -> vm_abc_ref_pu/1
  [vm_dq] -> Bus Generator1/2, RMS derivation1/1(dq)  "vm_dq"
  [ig_abc_pu] -> abc2dq0_norm/1
  [ig_abc_pu] -> " pu P/Q computation"/2(i_abc_pu)
  [vg_abc_pu] -> " pu P/Q computation"/1(v_abc_pu)
  [vg_abc_pu] -> PLL/1
  [Vg_rms] -> LPF1/1(In1)
  Constant7/1 -> Gain5/1
  From15/1 -> Divide5/2
  PLL/3 -> [w_PLL]
  PLL/2 -> [CosSinTheta]
  PLL/1 -> [Theta_PLL]
  Demux3/1 -> Divide3/1, Divide/1
  Divide4/1 -> Sum6/2
  Demux3/2 -> Divide4/1, Divide1/1
  Divide3/1 -> Sum5/2
  Demux2/1 -> Sum5/1
  Divide5/1 -> Divide1/2, Divide/2
  Divide/1 -> Sum6/3
  Mux3/1 -> norm1/1(In1)
  Sum6/1 -> Mux3/2
  Divide1/1 -> Sum5/3
  norm1/1(Out1) -> Goto18/1
  Constant2/1 -> Gain4/1
  Gain3/1 -> Demux2/1
  Demux2/2 -> Sum6/1
  From28/1 -> Gain3/1
  Sum5/1 -> Mux3/1
  Gain1/1 -> K_FRT/1
  [Iqref] -> Square1/1
  Square/1 -> Sum3/1
  Constant3/1 -> Square/1
  Sum3/1 -> Sqrt/1
  Sqrt/1 -> [Idmax]
  Square1/1 -> Sum3/2
  LPF1/1(Ref) -> PI_fw_init2/1
  Q_set/1 -> [Q_set]
  [Q] -> LPF2/1(In1)
  [Idmax] -> Mux2/1
  Constant5/1 -> Mux2/2
  Mux2/1 -> Inner Current Control/5(idq_max)
  [Iqref_PI] -> Add/2
  Add/1 -> Saturation2/1
  Constant4/1 -> Switch/2
  Constant9/1 -> Equal/2
  Constant8/1 -> Sum4/1
  Constant12/1 -> Sum4/3
  Divide2/1 -> Add/1
  [vd] -> Equal/1
  Data Type Conversion/1 -> Divide2/2
  Equal/1 -> Data Type Conversion/1
  Saturation1/1 -> Divide2/1
  K_FRT/1 -> Saturation1/1
  [V_RMS] -> Sum4/2
  Sum4/1 -> Gain1/1
  Saturation2/1 -> [Iqref]
  [igdq] -> Inner Current Control/2(ig_dq)
  [Idref_PI] -> Mux/1
  [Iqref] -> Mux/2
  [P] -> LPF/1(In1)
  P_set/1 -> [P_set]
  Bus Creator/1 -> Signal Conversion/1
  Bus Generator/1 -> [Vg]  "Vg"
  [CosSinTheta] -> abc2dq0_norm/2
  [CosSinTheta] -> CosSin_Delay/1
  abc2dq0_norm/2 -> Scope3/1, [igdq]  "ig_dq"
  ig_abc_pu/1 -> [ig_abc_pu]  "ig_abc_pu"
  " pu P/Q computation"/1(P) -> [P]  "P"
  vg_abc_pu/1 -> [vg_abc_pu]
  Inner Current Control/1(vm_dq_ref) -> [vm_dq]  "vm_dq"
  Constant15/1 -> Inner Current Control/3(w)
  [vm_dq] -> dq02abc_norm/1  "vm_dq"
  " pu P/Q computation"/2(Q) -> [Q]  "Q"
  dq02abc_norm/2 -> [vm_abc_ref_pu]  "vm_abc_pu"
  [w_PLL] -> Bus Creator/3  "f"
  [Q] -> Bus Creator/2  "Q"
  [P] -> Bus Creator/1  "P"
  Signal Conversion/1 -> m/1
  Mux/1 -> Inner Current Control/1(ig_dq_ref)
  Constant1/1 -> dq02abc_norm/2
  [vg_abc_pu] -> Bus Generator/1  "vg_abc_pu"
  RMS derivation1/1(rms) -> Bus Generator1/3  "Vg_RMS"
  Bus Generator1/1 -> [Vm]  "Vm"
  [Vm] -> Bus Creator/5  "Vm"
  [Vg] -> Bus Creator/6  "Vg"
  [Ig] -> Bus Creator/7  "Ig"
  [ig_abc_pu] -> Bus Generator2/1  "ig_abc_pu"
  Bus Generator2/1 -> [Ig]  "Ig"
  [igdq] -> RMS derivation2/1(dq), Bus Generator2/2  "idq_pu"
  RMS derivation2/1(rms) -> Bus Generator2/3  "Ig_RMS"
  Constant11/1 -> PI_fw_init/4
  Constant10/1 -> PI_fw_init/5
  PI_fw_init/1 -> Switch/1
  LPF2/1(Out1) -> PI_fw_init/1
  Constant18/1 -> PI_fw_init2/5
  Constant19/1 -> PI_fw_init2/4
  Switch/1 -> [Iqref_PI]
  LPF/1(Out1) -> PI_fw_init1/2
  [P_set] -> PI_fw_init1/1
  PI_fw_init1/1 -> [Idref_PI]

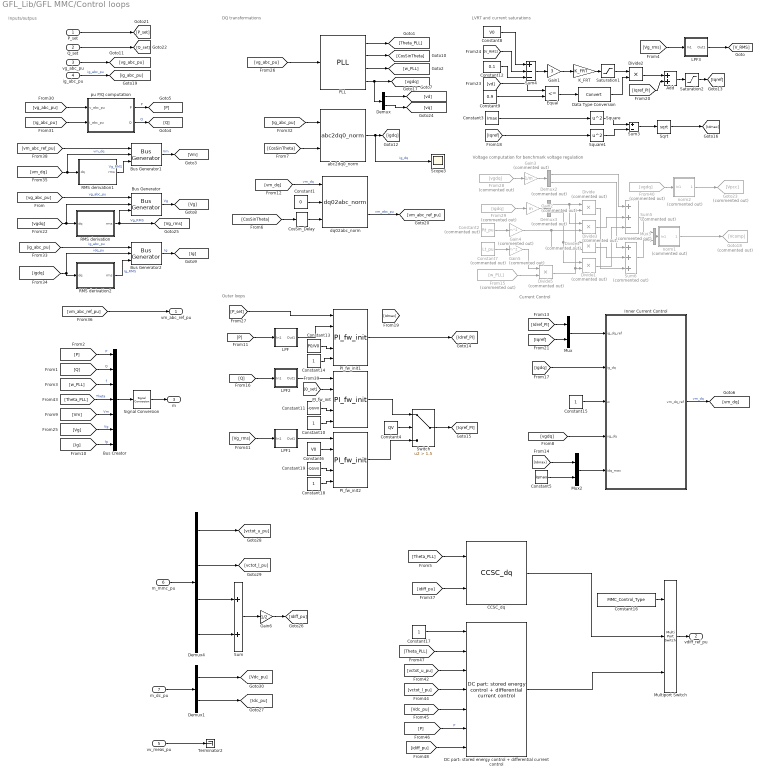
== system GFL_Lib/GFL MMC/Control loops ==
  note: Inputs/outpus
  note: DQ transformations
  note: Current Control
  note: Outer loops
  note: LVRT and current saturations
  note: Voltage computation for benchmark voltage regulation
  P_set : Inport
  Q_set : Inport  Port=2
  vg_abc_pu : Inport  Port=3
  ig_abc_pu : Inport  Port=4
  vv_meas_pu : Inport  Port=5
  m_mmc_pu : Inport  Port=6
  m_dc_pu : Inport  Port=7
  " pu P/Q computation" : Subsystem  DialogController=POWERSYS.PowerSysDialog
  Add : Sum
  Bus Creator : BusCreator  Inputs=7
  Bus Generator : Control_Lib/Bus Generator  Gpu=0
      settings: SourceProductName=VSC4SPS
  Bus Generator1 : Control_Lib/Bus Generator  Gpu=0
      settings: SourceProductName=VSC4SPS
  Bus Generator2 : Control_Lib/Bus Generator  Gpu=0
      settings: SourceProductName=VSC4SPS
  CCSC_dq : $bdroot/GFM_VC MMC/Control loops/CCSC_dq  SystemSampleTime=-1  Latency=0  AutoFrameSizeCalculation=off
  Constant1 : Constant  Value=0
  Constant{10,14..15,17..18} (5 alike) : Constant
  Constant11 : Constant  Value=-Q0/V0
  Constant12 : Constant  Value=0.1
  Constant13 : Constant  Value=P0/V0
  Constant16 : Constant  Value=MMC_Control_Type
  Constant19 : Constant  Value=-Q0/V0
  Constant2 : Constant  Commented=on  Value=Rt_pu
  Constant3 : Constant  Value=Imax
  Constant4 : Constant  Value=QV
  Constant5 : Constant  Value=Iqmax
  Constant6 : Constant  Value=V0
  Constant7 : Constant  Commented=on  Value=Lt_pu
  Constant8 : Constant  Value=V0
  Constant9 : Constant  Value=0.9
  CosSin_Delay : Control_Lib/CosSin_Delay  dTheta=wb*Output_Delay
      settings: SourceProductName=VSC4SPS
  DC part: stored energy control + differential current control : $bdroot/GFM_VC MMC/Control loops/DC part: stored energy control + differential current control  SystemSampleTime=-1  Latency=0  AutoFrameSizeCalculation=off
  Data Type Conversion : DataTypeConversion
  Demux : Demux  Outputs=[1 1]
  Demux1 : Demux  Outputs=2
  Demux2 : Demux  Commented=on  Outputs=2
  Demux3 : Demux  Commented=on  Outputs=2
  Demux4 : Demux  Outputs=[3 3 3 3]
  Divide{,1,3..5} (5 alike) : Product  Commented=on  Inputs=**
  Divide2 : Product  Inputs=**
  Equal : RelationalOperator  Operator=<=  OutDataTypeStr=boolean  RndMeth=Simplest
  From15 : From  Commented=on  GotoTag=w_PLL
  From28 : From  Commented=on  GotoTag=vgdq
  From29 : From  Commented=on  GotoTag=igdq
  From40 : From  Commented=on  GotoTag=vgdq
  Gain1 : Gain  Gain=3
  Gain2 : Gain  Commented=on  Gain=m
  Gain3 : Gain  Commented=on  Gain=1/m
  Gain4 : Gain  Commented=on  Gain=m^2
  Gain5 : Gain  Commented=on  Gain=m^2
  Gain6 : Gain  Gain=1/2
  Goto18 : Goto  Commented=on  GotoTag=Vcomp
  Goto23 : Goto  Commented=on  GotoTag=Vpcc
  Inner Current Control : Subsystem
  K_FRT : Gain  Gain=K_FRT
  LPF : Subsystem
  LPF1 : Subsystem
  LPF2 : Subsystem
  LPF3 : Subsystem
  Multiport Switch : MultiPortSwitch  Inputs=2
  Mux : Mux  Inputs=2
  Mux2 : Mux  Inputs=2
  Mux3 : Mux  Commented=on  Inputs=2
  PI_fw_init : Control_Lib/PI_fw_init  Kp=w_P/w_LPF  Ki=w_P
      settings: SourceProductName=VSC4SPS
  PI_fw_init1 : Control_Lib/PI_fw_init  Kp=w_P/w_LPF  Ki=w_P
      settings: SourceProductName=VSC4SPS
  PI_fw_init2 : Control_Lib/PI_fw_init  Kp=w_V/w_LPF  Ki=w_V
      settings: SourceProductName=VSC4SPS
  PLL : Control_Lib/PLL  fb=fb  wn_PLL=wn_PLL  zeta_PLL=zeta_PLL  Theta0=Theta0
      settings: SourceProductName=VSC4SPS
  RMS derivation : Subsystem
  RMS derivation1 : Subsystem
  RMS derivation2 : Subsystem
  Saturation1 : Saturate  UpperLimit=Imax  LowerLimit=-Imax
  Saturation2 : Saturate  UpperLimit=Imax  LowerLimit=-Imax
  Scope3 : Scope
  Signal Conversion : SignalConversion  OverrideOpt=off
  Sqrt : Sqrt  SaturateOnIntegerOverflow=on
  Square : Math  Operator=square  SaturateOnIntegerOverflow=on
  Square1 : Math  Operator=square  SaturateOnIntegerOverflow=on
  Sum : Sum
  Sum3 : Sum  Inputs=+-
  Sum4 : Sum  Inputs=+--
  Sum5 : Sum  Commented=on  Inputs=++-
  Sum6 : Sum  Commented=on  Inputs=+++
  Switch : Switch  Criteria=u2 > Threshold  Threshold=1.5
  Terminator2 : Terminator
  abc2dq0_norm : Control_Lib/abc2dq0_norm  referenceAxisMode=Reference axis at 90 degrees behind phase_a  baseUpdateGain=1/sqrt(3)
      settings: SourceProductName=VSC4SPS
  dq02abc_norm : Control_Lib/dq02abc_norm  referenceAxisMode=Reference axis at 90 degrees behind phase_a  baseUpdateGain=sqrt(3)
      settings: SourceProductName=VSC4SPS
  norm1 : Subsystem  Commented=on
  norm2 : Subsystem  Commented=on
  vm_abc_ref_pu : Outport  VectorParamsAs1DForOutWhenUnconnected=off
  vdiff_ref_pu : Outport  Port=2
  m : Outport  Port=3  VectorParamsAs1DForOutWhenUnconnected=off
  wires:
  Constant14/1 -> PI_fw_init1/5
  Constant13/1 -> PI_fw_init1/4
  [Vg_rms] -> LPF3/1(In1)
  LPF3/1(Out1) -> [V_RMS]
  CosSin_Delay/1 -> dq02abc_norm/3
  [Theta_PLL] -> Bus Creator/4  "Theta"
  RMS derivation/1(rms) -> Bus Generator/3, [Vg_rms]  "Vg_RMS"
  [vgdq] -> Bus Generator/2, RMS derivation/1(dq)
  Demux/2 -> [vq]
  Demux/1 -> [vd]
  PLL/4 -> [vgdq], Demux/1
  norm2/1(Out1) -> Goto23/1
  From40/1 -> norm2/1(In1)
  Gain4/1 -> Divide3/2, Divide4/2
  Gain5/1 -> Divide5/1
  Gain2/1 -> Demux3/1
  From29/1 -> Gain2/1
  [Q_set] -> PI_fw_init/2
  [vgdq] -> Inner Current Control/4(vg_dq)
  [vm_abc_ref_pu] -> Bus Generator1/1
  [vm_abc_ref_pu] -> vm_abc_ref_pu/1
  [vm_dq] -> Bus Generator1/2, RMS derivation1/1(dq)  "vm_dq"
  [ig_abc_pu] -> abc2dq0_norm/1
  [ig_abc_pu] -> " pu P/Q computation"/2(i_abc_pu)
  [vg_abc_pu] -> " pu P/Q computation"/1(v_abc_pu)
  [vg_abc_pu] -> PLL/1
  [Vg_rms] -> LPF1/1(In1)
  Constant7/1 -> Gain5/1
  From15/1 -> Divide5/2
  PLL/3 -> [w_PLL]
  PLL/2 -> [CosSinTheta]
  PLL/1 -> [Theta_PLL]
  Demux3/1 -> Divide3/1, Divide/1
  Divide4/1 -> Sum6/2
  Demux3/2 -> Divide4/1, Divide1/1
  Divide3/1 -> Sum5/2
  Demux2/1 -> Sum5/1
  Divide5/1 -> Divide1/2, Divide/2
  Divide/1 -> Sum6/3
  Mux3/1 -> norm1/1(In1)
  Sum6/1 -> Mux3/2
  Divide1/1 -> Sum5/3
  norm1/1(Out1) -> Goto18/1
  Constant2/1 -> Gain4/1
  Gain3/1 -> Demux2/1
  Demux2/2 -> Sum6/1
  From28/1 -> Gain3/1
  Sum5/1 -> Mux3/1
  Gain1/1 -> K_FRT/1
  [Iqref] -> Square1/1
  Square/1 -> Sum3/1
  Constant3/1 -> Square/1
  Sum3/1 -> Sqrt/1
  Sqrt/1 -> [Idmax]
  Square1/1 -> Sum3/2
  Q_set/1 -> [Q_set]
  [Q] -> LPF2/1(In1)
  [Idmax] -> Mux2/1
  Constant5/1 -> Mux2/2
  Mux2/1 -> Inner Current Control/5(idq_max)
  [Iqref_PI] -> Add/2
  Add/1 -> Saturation2/1
  Constant4/1 -> Switch/2
  Constant9/1 -> Equal/2
  Constant8/1 -> Sum4/1
  Constant12/1 -> Sum4/3
  Divide2/1 -> Add/1
  [vd] -> Equal/1
  Data Type Conversion/1 -> Divide2/2
  Equal/1 -> Data Type Conversion/1
  Saturation1/1 -> Divide2/1
  K_FRT/1 -> Saturation1/1
  [V_RMS] -> Sum4/2
  Sum4/1 -> Gain1/1
  Saturation2/1 -> [Iqref]
  [igdq] -> Inner Current Control/2(ig_dq)
  [Idref_PI] -> Mux/1
  [Iqref] -> Mux/2
  [P] -> LPF/1(In1)
  P_set/1 -> [P_set]
  Bus Creator/1 -> Signal Conversion/1
  Bus Generator/1 -> [Vg]  "Vg"
  [CosSinTheta] -> abc2dq0_norm/2
  [CosSinTheta] -> CosSin_Delay/1
  abc2dq0_norm/2 -> Scope3/1, [igdq]  "ig_dq"
  ig_abc_pu/1 -> [ig_abc_pu]  "ig_abc_pu"
  " pu P/Q computation"/1(P) -> [P]  "P"
  vg_abc_pu/1 -> [vg_abc_pu]
  Inner Current Control/1(vm_dq_ref) -> [vm_dq]  "vm_dq"
  Constant15/1 -> Inner Current Control/3(w)
  [vm_dq] -> dq02abc_norm/1  "vm_dq"
  " pu P/Q computation"/2(Q) -> [Q]  "Q"
  dq02abc_norm/2 -> [vm_abc_ref_pu]  "vm_abc_pu"
  [w_PLL] -> Bus Creator/3  "f"
  [Q] -> Bus Creator/2  "Q"
  [P] -> Bus Creator/1  "P"
  Signal Conversion/1 -> m/1
  Mux/1 -> Inner Current Control/1(ig_dq_ref)
  Constant1/1 -> dq02abc_norm/2
  [vg_abc_pu] -> Bus Generator/1  "vg_abc_pu"
  RMS derivation1/1(rms) -> Bus Generator1/3  "Vg_RMS"
  Bus Generator1/1 -> [Vm]  "Vm"
  [Vm] -> Bus Creator/5  "Vm"
  [Vg] -> Bus Creator/6  "Vg"
  [Ig] -> Bus Creator/7  "Ig"
  [ig_abc_pu] -> Bus Generator2/1  "ig_abc_pu"
  Bus Generator2/1 -> [Ig]  "Ig"
  [igdq] -> RMS derivation2/1(dq), Bus Generator2/2  "idq_pu"
  RMS derivation2/1(rms) -> Bus Generator2/3  "Ig_RMS"
  Constant11/1 -> PI_fw_init/4
  Constant10/1 -> PI_fw_init/5
  PI_fw_init/1 -> Switch/1
  LPF2/1(Out1) -> PI_fw_init/1
  Constant18/1 -> PI_fw_init2/5
  Constant19/1 -> PI_fw_init2/4
  PI_fw_init2/1 -> Switch/3
  Switch/1 -> [Iqref_PI]
  LPF/1(Out1) -> PI_fw_init1/2
  [P_set] -> PI_fw_init1/1
  PI_fw_init1/1 -> [Idref_PI]
  [P] -> DC part: stored energy control + differential current control/6  "P"
  [vctot_l_pu] -> DC part: stored energy control + differential current control/4
  vv_meas_pu/1 -> Terminator2/1
  Demux4/3 -> Sum/1
  CCSC_dq/1 -> Multiport Switch/2
  Demux4/4 -> Sum/2
  [vctot_u_pu] -> DC part: stored energy control + differential current control/3
  [Vdc_pu] -> DC part: stored energy control + differential current control/5
  m_dc_pu/1 -> Demux1/1
  Sum/1 -> Gain6/1
  Constant16/1 -> Multiport Switch/1
  [Theta_PLL] -> DC part: stored energy control + differential current control/2
  [Theta_PLL] -> CCSC_dq/1
  Constant17/1 -> DC part: stored energy control + differential current control/1
  Demux1/1 -> [Vdc_pu]
  DC part: stored energy control + differential current control/1 -> Multiport Switch/3
  [idiff_pu] -> DC part: stored energy control + differential current control/7
  m_mmc_pu/1 -> Demux4/1
  Demux4/2 -> [vctot_l_pu]
  Multiport Switch/1 -> vdiff_ref_pu/1
  Demux1/2 -> [Idc_pu]
  Demux4/1 -> [vctot_u_pu]
  [idiff_pu] -> CCSC_dq/2
  Gain6/1 -> [idiff_pu]
  LPF1/1(Out1) -> PI_fw_init2/1
  Constant6/1 -> PI_fw_init2/2
